simulink model "estimatetransform"  (R2019b)
settings: Solver=VariableStepAuto  StartTime=0.0  StopTime=10.0  RelTol=1e-3
values from neighbouring files (symbols this model uses):
  matchedPtsDistorted = [ [550.2,93.45], ... (first row only)    [matchpoints.m]    (also in points.m)
  matchedPtsOriginal = [ [810.7,115.3], ... (first row only)    [matchpoints.m]    (also in points.m)
libraries: visiongeotforms x1
settings Model: Creator=zacefron  LastModifiedBy=zacefron

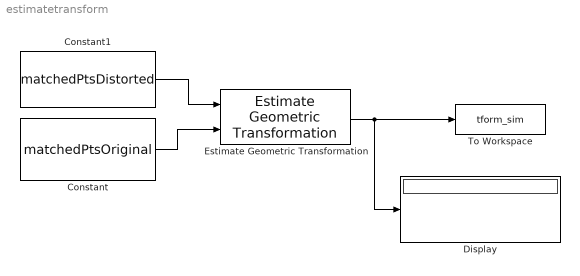
== system estimatetransform ==
  Constant : Constant  Value=matchedPtsOriginal
  Constant1 : Constant  Value=matchedPtsDistorted
  Display : Display
      settings: Decimation=3
  Estimate Geometric Transformation : visiongeotforms/Estimate Geometric Transformation  tformType=Affine  isRandomSampling=off  algMethod=Random Sample Consensus (RANSAC)  distanceAlg=2.5  distanceGeo=2.5  numMethod=Specified value  sampleNum=500  desiredConfidence=99  maxSampleNum=1000  isStopSampling=off  percentStop=75  isRefineTForm=off  isReleaseMode=on  isOutputInlier=off  outDT4IntInput=Obsolete10a  outDT4IntInputActive=Double  isVarSizeAllowed=on
      settings: SourceProductName=Computer Vision Toolbox  SourceProductBaseCode=VP
  To Workspace : ToWorkspace  VariableName=tform_sim  SampleTime=-1
      settings: Save2DSignal=2-D array (concatenate along first dimension)
  wires:
  Estimate Geometric Transformation/1 -> To Workspace/1, Display/1
  Constant1/1 -> Estimate Geometric Transformation/1
  Constant/1 -> Estimate Geometric Transformation/2
